simulink model "lookup_nD_TestGen21"  (R2017b)
settings: Solver=FixedStepDiscrete  StartTime=0.0  StopTime=10.0  RelTol=1e-3
model workspace (MAT data in the model file):
  LUTObjLKnD21 = Simulink.LookupTable
  LUTObjLKnD21.Table = Simulink.lookuptable.Table
  LUTObjLKnD21.Table.Value = reshape([4 16 10 4 16 10 5 19 18 5 19 18 6 20 23 6 20 23 7 21 24 7 21 24 8 22 25 8 22 25 4 16 10 4 16 10 5 19 18 5 19 18 6 20 23 6 20 23 7 21 24 7 21 24 8 22 25 8 22 25], [2 5 3 2])
  LUTObjLKnD21.Table.Dimensions = [2 5 3 2]
  LUTObjLKnD21.Table.DataType = 'double'
  LUTObjLKnD21.Table.FieldName = 'Table'
  LUTObjLKnD21.Breakpoints(1) = Simulink.lookuptable.Breakpoint
  LUTObjLKnD21.Breakpoints(1).Value = [15.6417382213; 44.1993458275]
  LUTObjLKnD21.Breakpoints(1).TunableSizeName = 'N1'
  LUTObjLKnD21.Breakpoints(1).Dimensions = [2 1]
  LUTObjLKnD21.Breakpoints(1).DataType = 'double'
  LUTObjLKnD21.Breakpoints(1).FieldName = 'BP1'
  LUTObjLKnD21.Breakpoints(2) = Simulink.lookuptable.Breakpoint
  LUTObjLKnD21.Breakpoints(2).Value = [7.9047999552; 49.0363144642; 53.4335142259; 57.8317081468; 58.4949480026]
  LUTObjLKnD21.Breakpoints(2).TunableSizeName = 'N2'
  LUTObjLKnD21.Breakpoints(2).Dimensions = [5 1]
  LUTObjLKnD21.Breakpoints(2).DataType = 'double'
  LUTObjLKnD21.Breakpoints(2).FieldName = 'BP2'
  LUTObjLKnD21.Breakpoints(3) = Simulink.lookuptable.Breakpoint
  LUTObjLKnD21.Breakpoints(3).Value = [69.8081328429; 102.684618613; 125.878045002]
  LUTObjLKnD21.Breakpoints(3).TunableSizeName = 'N3'
  LUTObjLKnD21.Breakpoints(3).Dimensions = [3 1]
  LUTObjLKnD21.Breakpoints(3).DataType = 'double'
  LUTObjLKnD21.Breakpoints(3).FieldName = 'BP3'
  LUTObjLKnD21.Breakpoints(4) = Simulink.lookuptable.Breakpoint
  LUTObjLKnD21.Breakpoints(4).Value = [57.8643810111; 102.455871762]
  LUTObjLKnD21.Breakpoints(4).TunableSizeName = 'N4'
  LUTObjLKnD21.Breakpoints(4).Dimensions = [2 1]
  LUTObjLKnD21.Breakpoints(4).DataType = 'double'
  LUTObjLKnD21.Breakpoints(4).FieldName = 'BP4'
  LUTObjLKnD21.SupportTunableSize = 0
  LUTObjLKnD21.StructTypeInfo = Simulink.lookuptable.StructTypeInfo
  LUTObjLKnD21.StructTypeInfo.Name = 'LUT'
  LUTObjLKnD21.StructTypeInfo.DataScope = 'Auto'
settings Model: Creator=ktrinh  LastModifiedBy=ktrinh
settings DebuggingCC: ParameterOverflowMsg=none

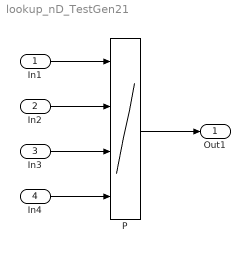
== system lookup_nD_TestGen21 ==
  In1 : Inport  OutMin=0  OutMax=127  PortDimensions=1
  In2 : Inport  Port=2  OutMin=0  OutMax=127
  In3 : Inport  Port=3  OutMin=0  OutMax=127
  In4 : Inport  Port=4  OutMin=0  OutMax=127
  P : Lookup_n-D  NumberOfTableDimensions=4  DataSpecification=Lookup table object  LookupTableObject=LUTObjLKnD21  BreakpointsForDimension3=[5, 7]  Table=reshape(repmat([4 5 6;16 19 20;10 18 23],1,2),[3,3,2])  InterpMethod=Nearest  ExtrapMethod=Clip  InternalRulePriority=Speed  OutDataTypeStr=double  RndMeth=Ceiling  SaturateOnIntegerOverflow=on  InputSameDT=on
  Out1 : Outport
  wires:
  In1/1 -> P/1
  In2/1 -> P/2
  In3/1 -> P/3
  In4/1 -> P/4
  P/1 -> Out1/1
